simulink model "main1"  (Simulink 10.0)
settings: Solver=ode45  StartTime=0.0  StopTime=0.5  RelTol=1e-3  EnableMultiTasking=on
undefined symbols (not defined in the file): D1, Delta, DiscIntNeverNeededParam, Hydride, Metal, Nickel
libraries: elec_lib x216, powerlib x83, fl_lib x9, powerlib_extras x8, simulink x3, nesl_utility x2, electricdrivelib x1
(part 2 of 2)

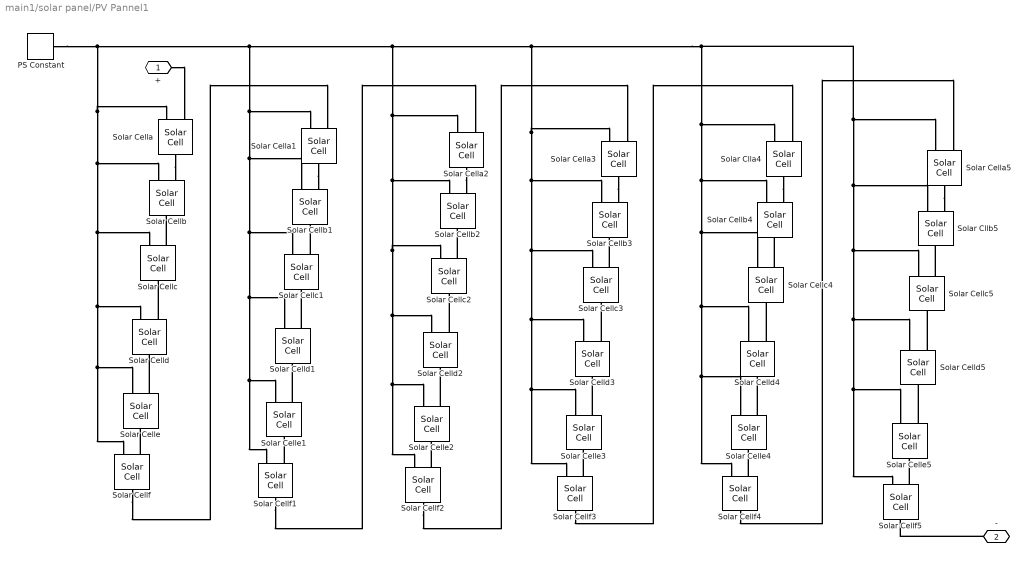
== system main1/solar panel/PV Pannel1 ==
  PS Constant : fl_lib/Physical Signals/Sources/PS Constant  SystemSampleTime=-1  constant=687  LocalVarLogging=[]
  Solar Cella{,1..3,5} (5 alike) : elec_lib/Sources/Solar Cell  SystemSampleTime=-1  prm=1  Isc=2.54 A  Voc=21.8 V  Is=1e-6 A  Is2=0 A  Iph=7.34 A  Ir0=1000 W/m^2  ec=1.6  N2=2  Rs=5.1e-3 Ohm  Rp=Inf Ohm  TIPH1=0.65e-3 1/K  EG=1.12 eV  TXIS1=3  TXIS2=3  TRS1=0  TRP1=0  TFIXED=25 C  Tmeas=25 C  LocalVarLogging=[]
      settings: SourceProductName=Simscape Electrical  SourceProductBaseCode=PS
  Solar Cellb{,1..4} (5 alike) : elec_lib/Sources/Solar Cell  SystemSampleTime=-1  prm=1  Isc=2.54 A  Voc=21.8 V  Is=1e-6 A  Is2=0 A  Iph=7.34 A  Ir0=1000 W/m^2  ec=1.6  N2=2  Rs=5.1e-3 Ohm  Rp=Inf Ohm  TIPH1=0.65e-3 1/K  EG=1.12 eV  TXIS1=3  TXIS2=3  TRS1=0  TRP1=0  TFIXED=25 C  Tmeas=25 C  LocalVarLogging=[]
      settings: SourceProductName=Simscape Electrical  SourceProductBaseCode=PS
  Solar Cellc{,1..5} (6 alike) : elec_lib/Sources/Solar Cell  SystemSampleTime=-1  prm=1  Isc=2.54 A  Voc=21.8 V  Is=1e-6 A  Is2=0 A  Iph=7.34 A  Ir0=1000 W/m^2  ec=1.6  N2=2  Rs=5.1e-3 Ohm  Rp=Inf Ohm  TIPH1=0.65e-3 1/K  EG=1.12 eV  TXIS1=3  TXIS2=3  TRS1=0  TRP1=0  TFIXED=25 C  Tmeas=25 C  LocalVarLogging=[]
      settings: SourceProductName=Simscape Electrical  SourceProductBaseCode=PS
  Solar Celld{,1..5} (6 alike) : elec_lib/Sources/Solar Cell  SystemSampleTime=-1  prm=1  Isc=2.54 A  Voc=21.8 V  Is=1e-6 A  Is2=0 A  Iph=7.34 A  Ir0=1000 W/m^2  ec=1.6  N2=2  Rs=5.1e-3 Ohm  Rp=Inf Ohm  TIPH1=0.65e-3 1/K  EG=1.12 eV  TXIS1=3  TXIS2=3  TRS1=0  TRP1=0  TFIXED=25 C  Tmeas=25 C  LocalVarLogging=[]
      settings: SourceProductName=Simscape Electrical  SourceProductBaseCode=PS
  Solar Celle{,1..5} (6 alike) : elec_lib/Sources/Solar Cell  SystemSampleTime=-1  prm=1  Isc=2.54 A  Voc=21.8 V  Is=1e-6 A  Is2=0 A  Iph=7.34 A  Ir0=1000 W/m^2  ec=1.6  N2=2  Rs=5.1e-3 Ohm  Rp=Inf Ohm  TIPH1=0.65e-3 1/K  EG=1.12 eV  TXIS1=3  TXIS2=3  TRS1=0  TRP1=0  TFIXED=25 C  Tmeas=25 C  LocalVarLogging=[]
      settings: SourceProductName=Simscape Electrical  SourceProductBaseCode=PS
  Solar Cellf{,1..5} (6 alike) : elec_lib/Sources/Solar Cell  SystemSampleTime=-1  prm=1  Isc=2.54 A  Voc=21.8 V  Is=1e-6 A  Is2=0 A  Iph=7.34 A  Ir0=1000 W/m^2  ec=1.6  N2=2  Rs=5.1e-3 Ohm  Rp=Inf Ohm  TIPH1=0.65e-3 1/K  EG=1.12 eV  TXIS1=3  TXIS2=3  TRS1=0  TRP1=0  TFIXED=25 C  Tmeas=25 C  LocalVarLogging=[]
      settings: SourceProductName=Simscape Electrical  SourceProductBaseCode=PS
  Solar Clla4 : elec_lib/Sources/Solar Cell  SystemSampleTime=-1  prm=1  Isc=2.54 A  Voc=21.8 V  Is=1e-6 A  Is2=0 A  Iph=7.34 A  Ir0=1000 W/m^2  ec=1.6  N2=2  Rs=5.1e-3 Ohm  Rp=Inf Ohm  TIPH1=0.65e-3 1/K  EG=1.12 eV  TXIS1=3  TXIS2=3  TRS1=0  TRP1=0  TFIXED=25 C  Tmeas=25 C  LocalVarLogging=[]
      settings: SourceProductName=Simscape Electrical  SourceProductBaseCode=PS
  Solar Cllb5 : elec_lib/Sources/Solar Cell  SystemSampleTime=-1  prm=1  Isc=2.54 A  Voc=21.8 V  Is=1e-6 A  Is2=0 A  Iph=7.34 A  Ir0=1000 W/m^2  ec=1.6  N2=2  Rs=5.1e-3 Ohm  Rp=Inf Ohm  TIPH1=0.65e-3 1/K  EG=1.12 eV  TXIS1=3  TXIS2=3  TRS1=0  TRP1=0  TFIXED=25 C  Tmeas=25 C  LocalVarLogging=[]
      settings: SourceProductName=Simscape Electrical  SourceProductBaseCode=PS
  + : PMIOPort  Side=Left
  - : PMIOPort  Port=2  Side=Left
  connections:
  -/RConn1 -- Solar Cellf5/RConn1
  +/RConn1 -- Solar Cella/LConn2
  Solar Cella3/LConn1 -- Solar Cellb3/LConn1 -- Solar Cellc3/LConn1 -- Solar Celld3/LConn1 -- Solar Celle3/LConn1 -- Solar Cellf3/LConn1 -- Solar Celle2/LConn1 -- Solar Cellf2/LConn1 -- Solar Celld2/LConn1 -- Solar Cellc2/LConn1 -- Solar Cellb2/LConn1 -- Solar Cella2/LConn1 -- Solar Cella1/LConn1 -- Solar Cellb1/LConn1 -- Solar Cellc1/LConn1 -- Solar Celld1/LConn1 -- Solar Celle1/LConn1 -- Solar Cellf1/LConn1 -- Solar Cella/LConn1 -- Solar Cellb/LConn1 -- Solar Cellc/LConn1 -- Solar Celld/LConn1 -- Solar Celle/LConn1 -- Solar Cellf/LConn1 -- PS Constant/RConn1 -- Solar Celle5/LConn1 -- Solar Cellf5/LConn1 -- Solar Celld5/LConn1 -- Solar Cellc5/LConn1 -- Solar Cllb5/LConn1 -- Solar Cella5/LConn1 -- Solar Clla4/LConn1 -- Solar Cellb4/LConn1 -- Solar Cellc4/LConn1 -- Solar Celld4/LConn1 -- Solar Celle4/LConn1 -- Solar Cellf4/LConn1
  Solar Cellf4/RConn1 -- Solar Cella5/LConn2
  Solar Cellf3/RConn1 -- Solar Clla4/LConn2
  Solar Cellf2/RConn1 -- Solar Cella3/LConn2
  Solar Cellf1/RConn1 -- Solar Cella2/LConn2
  Solar Cellf/RConn1 -- Solar Cella1/LConn2
  Solar Cellf5/LConn2 -- Solar Celle5/RConn1
  Solar Celle5/LConn2 -- Solar Celld5/RConn1
  Solar Celld5/LConn2 -- Solar Cellc5/RConn1
  Solar Cellc5/LConn2 -- Solar Cllb5/RConn1
  Solar Cella5/RConn1 -- Solar Cllb5/LConn2
  Solar Cellf4/LConn2 -- Solar Celle4/RConn1
  Solar Celle4/LConn2 -- Solar Celld4/RConn1
  Solar Celld4/LConn2 -- Solar Cellc4/RConn1
  Solar Cellc4/LConn2 -- Solar Cellb4/RConn1
  Solar Clla4/RConn1 -- Solar Cellb4/LConn2
  Solar Cellf3/LConn2 -- Solar Celle3/RConn1
  Solar Celle3/LConn2 -- Solar Celld3/RConn1
  Solar Celld3/LConn2 -- Solar Cellc3/RConn1
  Solar Cellc3/LConn2 -- Solar Cellb3/RConn1
  Solar Cella3/RConn1 -- Solar Cellb3/LConn2
  Solar Cellf2/LConn2 -- Solar Celle2/RConn1
  Solar Celle2/LConn2 -- Solar Celld2/RConn1
  Solar Celld2/LConn2 -- Solar Cellc2/RConn1
  Solar Cellc2/LConn2 -- Solar Cellb2/RConn1
  Solar Cella2/RConn1 -- Solar Cellb2/LConn2
  Solar Cellf1/LConn2 -- Solar Celle1/RConn1
  Solar Celle1/LConn2 -- Solar Celld1/RConn1
  Solar Celld1/LConn2 -- Solar Cellc1/RConn1
  Solar Cellc1/LConn2 -- Solar Cellb1/RConn1
  Solar Cella1/RConn1 -- Solar Cellb1/LConn2
  Solar Cellf/LConn2 -- Solar Celle/RConn1
  Solar Celle/LConn2 -- Solar Celld/RConn1
  Solar Celld/LConn2 -- Solar Cellc/RConn1
  Solar Cellc/LConn2 -- Solar Cellb/RConn1
  Solar Cella/RConn1 -- Solar Cellb/LConn2

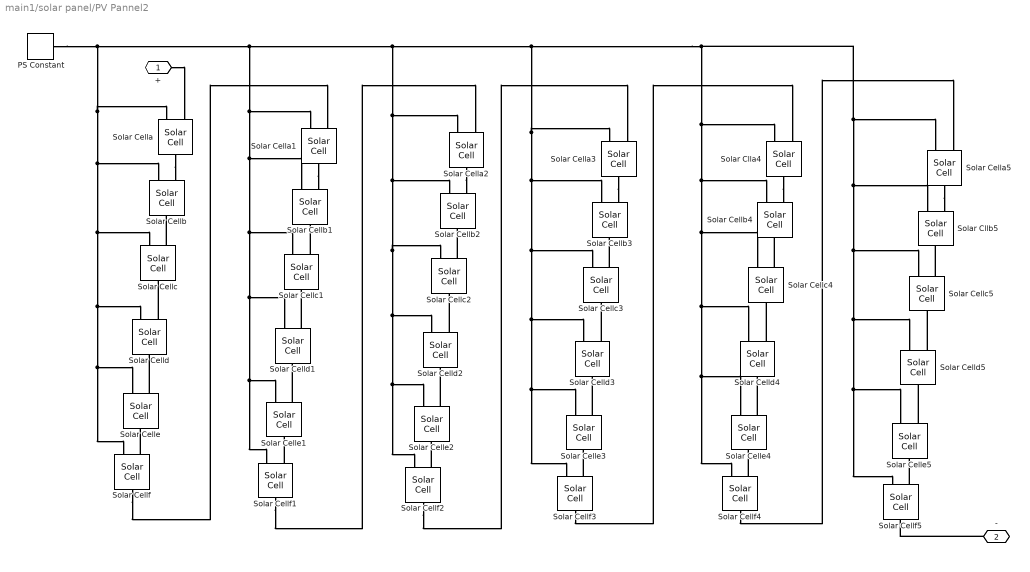
== system main1/solar panel/PV Pannel2 ==
  PS Constant : fl_lib/Physical Signals/Sources/PS Constant  SystemSampleTime=-1  constant=687  LocalVarLogging=[]
  Solar Cella{,1..3,5} (5 alike) : elec_lib/Sources/Solar Cell  SystemSampleTime=-1  prm=1  Isc=2.54 A  Voc=21.8 V  Is=1e-6 A  Is2=0 A  Iph=7.34 A  Ir0=1000 W/m^2  ec=1.6  N2=2  Rs=5.1e-3 Ohm  Rp=Inf Ohm  TIPH1=0.65e-3 1/K  EG=1.12 eV  TXIS1=3  TXIS2=3  TRS1=0  TRP1=0  TFIXED=25 C  Tmeas=25 C  LocalVarLogging=[]
      settings: SourceProductName=Simscape Electrical  SourceProductBaseCode=PS
  Solar Cellb{,1..4} (5 alike) : elec_lib/Sources/Solar Cell  SystemSampleTime=-1  prm=1  Isc=2.54 A  Voc=21.8 V  Is=1e-6 A  Is2=0 A  Iph=7.34 A  Ir0=1000 W/m^2  ec=1.6  N2=2  Rs=5.1e-3 Ohm  Rp=Inf Ohm  TIPH1=0.65e-3 1/K  EG=1.12 eV  TXIS1=3  TXIS2=3  TRS1=0  TRP1=0  TFIXED=25 C  Tmeas=25 C  LocalVarLogging=[]
      settings: SourceProductName=Simscape Electrical  SourceProductBaseCode=PS
  Solar Cellc{,1..5} (6 alike) : elec_lib/Sources/Solar Cell  SystemSampleTime=-1  prm=1  Isc=2.54 A  Voc=21.8 V  Is=1e-6 A  Is2=0 A  Iph=7.34 A  Ir0=1000 W/m^2  ec=1.6  N2=2  Rs=5.1e-3 Ohm  Rp=Inf Ohm  TIPH1=0.65e-3 1/K  EG=1.12 eV  TXIS1=3  TXIS2=3  TRS1=0  TRP1=0  TFIXED=25 C  Tmeas=25 C  LocalVarLogging=[]
      settings: SourceProductName=Simscape Electrical  SourceProductBaseCode=PS
  Solar Celld{,1..5} (6 alike) : elec_lib/Sources/Solar Cell  SystemSampleTime=-1  prm=1  Isc=2.54 A  Voc=21.8 V  Is=1e-6 A  Is2=0 A  Iph=7.34 A  Ir0=1000 W/m^2  ec=1.6  N2=2  Rs=5.1e-3 Ohm  Rp=Inf Ohm  TIPH1=0.65e-3 1/K  EG=1.12 eV  TXIS1=3  TXIS2=3  TRS1=0  TRP1=0  TFIXED=25 C  Tmeas=25 C  LocalVarLogging=[]
      settings: SourceProductName=Simscape Electrical  SourceProductBaseCode=PS
  Solar Celle{,1..5} (6 alike) : elec_lib/Sources/Solar Cell  SystemSampleTime=-1  prm=1  Isc=2.54 A  Voc=21.8 V  Is=1e-6 A  Is2=0 A  Iph=7.34 A  Ir0=1000 W/m^2  ec=1.6  N2=2  Rs=5.1e-3 Ohm  Rp=Inf Ohm  TIPH1=0.65e-3 1/K  EG=1.12 eV  TXIS1=3  TXIS2=3  TRS1=0  TRP1=0  TFIXED=25 C  Tmeas=25 C  LocalVarLogging=[]
      settings: SourceProductName=Simscape Electrical  SourceProductBaseCode=PS
  Solar Cellf{,1..5} (6 alike) : elec_lib/Sources/Solar Cell  SystemSampleTime=-1  prm=1  Isc=2.54 A  Voc=21.8 V  Is=1e-6 A  Is2=0 A  Iph=7.34 A  Ir0=1000 W/m^2  ec=1.6  N2=2  Rs=5.1e-3 Ohm  Rp=Inf Ohm  TIPH1=0.65e-3 1/K  EG=1.12 eV  TXIS1=3  TXIS2=3  TRS1=0  TRP1=0  TFIXED=25 C  Tmeas=25 C  LocalVarLogging=[]
      settings: SourceProductName=Simscape Electrical  SourceProductBaseCode=PS
  Solar Clla4 : elec_lib/Sources/Solar Cell  SystemSampleTime=-1  prm=1  Isc=2.54 A  Voc=21.8 V  Is=1e-6 A  Is2=0 A  Iph=7.34 A  Ir0=1000 W/m^2  ec=1.6  N2=2  Rs=5.1e-3 Ohm  Rp=Inf Ohm  TIPH1=0.65e-3 1/K  EG=1.12 eV  TXIS1=3  TXIS2=3  TRS1=0  TRP1=0  TFIXED=25 C  Tmeas=25 C  LocalVarLogging=[]
      settings: SourceProductName=Simscape Electrical  SourceProductBaseCode=PS
  Solar Cllb5 : elec_lib/Sources/Solar Cell  SystemSampleTime=-1  prm=1  Isc=2.54 A  Voc=21.8 V  Is=1e-6 A  Is2=0 A  Iph=7.34 A  Ir0=1000 W/m^2  ec=1.6  N2=2  Rs=5.1e-3 Ohm  Rp=Inf Ohm  TIPH1=0.65e-3 1/K  EG=1.12 eV  TXIS1=3  TXIS2=3  TRS1=0  TRP1=0  TFIXED=25 C  Tmeas=25 C  LocalVarLogging=[]
      settings: SourceProductName=Simscape Electrical  SourceProductBaseCode=PS
  + : PMIOPort  Side=Left
  - : PMIOPort  Port=2  Side=Left
  connections:
  -/RConn1 -- Solar Cellf5/RConn1
  +/RConn1 -- Solar Cella/LConn2
  Solar Cella3/LConn1 -- Solar Cellb3/LConn1 -- Solar Cellc3/LConn1 -- Solar Celld3/LConn1 -- Solar Celle3/LConn1 -- Solar Cellf3/LConn1 -- Solar Celle2/LConn1 -- Solar Cellf2/LConn1 -- Solar Celld2/LConn1 -- Solar Cellc2/LConn1 -- Solar Cellb2/LConn1 -- Solar Cella2/LConn1 -- Solar Cella1/LConn1 -- Solar Cellb1/LConn1 -- Solar Cellc1/LConn1 -- Solar Celld1/LConn1 -- Solar Celle1/LConn1 -- Solar Cellf1/LConn1 -- Solar Cella/LConn1 -- Solar Cellb/LConn1 -- Solar Cellc/LConn1 -- Solar Celld/LConn1 -- Solar Celle/LConn1 -- Solar Cellf/LConn1 -- PS Constant/RConn1 -- Solar Celle5/LConn1 -- Solar Cellf5/LConn1 -- Solar Celld5/LConn1 -- Solar Cellc5/LConn1 -- Solar Cllb5/LConn1 -- Solar Cella5/LConn1 -- Solar Clla4/LConn1 -- Solar Cellb4/LConn1 -- Solar Cellc4/LConn1 -- Solar Celld4/LConn1 -- Solar Celle4/LConn1 -- Solar Cellf4/LConn1
  Solar Cellf4/RConn1 -- Solar Cella5/LConn2
  Solar Cellf3/RConn1 -- Solar Clla4/LConn2
  Solar Cellf2/RConn1 -- Solar Cella3/LConn2
  Solar Cellf1/RConn1 -- Solar Cella2/LConn2
  Solar Cellf/RConn1 -- Solar Cella1/LConn2
  Solar Cellf5/LConn2 -- Solar Celle5/RConn1
  Solar Celle5/LConn2 -- Solar Celld5/RConn1
  Solar Celld5/LConn2 -- Solar Cellc5/RConn1
  Solar Cellc5/LConn2 -- Solar Cllb5/RConn1
  Solar Cella5/RConn1 -- Solar Cllb5/LConn2
  Solar Cellf4/LConn2 -- Solar Celle4/RConn1
  Solar Celle4/LConn2 -- Solar Celld4/RConn1
  Solar Celld4/LConn2 -- Solar Cellc4/RConn1
  Solar Cellc4/LConn2 -- Solar Cellb4/RConn1
  Solar Clla4/RConn1 -- Solar Cellb4/LConn2
  Solar Cellf3/LConn2 -- Solar Celle3/RConn1
  Solar Celle3/LConn2 -- Solar Celld3/RConn1
  Solar Celld3/LConn2 -- Solar Cellc3/RConn1
  Solar Cellc3/LConn2 -- Solar Cellb3/RConn1
  Solar Cella3/RConn1 -- Solar Cellb3/LConn2
  Solar Cellf2/LConn2 -- Solar Celle2/RConn1
  Solar Celle2/LConn2 -- Solar Celld2/RConn1
  Solar Celld2/LConn2 -- Solar Cellc2/RConn1
  Solar Cellc2/LConn2 -- Solar Cellb2/RConn1
  Solar Cella2/RConn1 -- Solar Cellb2/LConn2
  Solar Cellf1/LConn2 -- Solar Celle1/RConn1
  Solar Celle1/LConn2 -- Solar Celld1/RConn1
  Solar Celld1/LConn2 -- Solar Cellc1/RConn1
  Solar Cellc1/LConn2 -- Solar Cellb1/RConn1
  Solar Cella1/RConn1 -- Solar Cellb1/LConn2
  Solar Cellf/LConn2 -- Solar Celle/RConn1
  Solar Celle/LConn2 -- Solar Celld/RConn1
  Solar Celld/LConn2 -- Solar Cellc/RConn1
  Solar Cellc/LConn2 -- Solar Cellb/RConn1
  Solar Cella/RConn1 -- Solar Cellb/LConn2

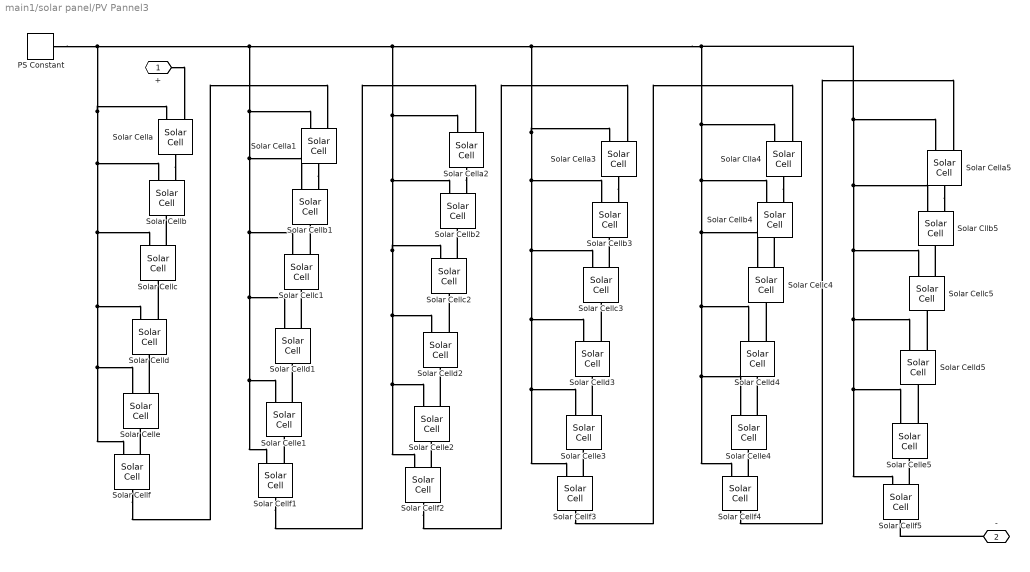
== system main1/solar panel/PV Pannel3 ==
  PS Constant : fl_lib/Physical Signals/Sources/PS Constant  SystemSampleTime=-1  constant=687  LocalVarLogging=[]
  Solar Cella{,1..3,5} (5 alike) : elec_lib/Sources/Solar Cell  SystemSampleTime=-1  prm=1  Isc=2.54 A  Voc=21.8 V  Is=1e-6 A  Is2=0 A  Iph=7.34 A  Ir0=1000 W/m^2  ec=1.6  N2=2  Rs=5.1e-3 Ohm  Rp=Inf Ohm  TIPH1=0.65e-3 1/K  EG=1.12 eV  TXIS1=3  TXIS2=3  TRS1=0  TRP1=0  TFIXED=25 C  Tmeas=25 C  LocalVarLogging=[]
      settings: SourceProductName=Simscape Electrical  SourceProductBaseCode=PS
  Solar Cellb{,1..4} (5 alike) : elec_lib/Sources/Solar Cell  SystemSampleTime=-1  prm=1  Isc=2.54 A  Voc=21.8 V  Is=1e-6 A  Is2=0 A  Iph=7.34 A  Ir0=1000 W/m^2  ec=1.6  N2=2  Rs=5.1e-3 Ohm  Rp=Inf Ohm  TIPH1=0.65e-3 1/K  EG=1.12 eV  TXIS1=3  TXIS2=3  TRS1=0  TRP1=0  TFIXED=25 C  Tmeas=25 C  LocalVarLogging=[]
      settings: SourceProductName=Simscape Electrical  SourceProductBaseCode=PS
  Solar Cellc{,1..5} (6 alike) : elec_lib/Sources/Solar Cell  SystemSampleTime=-1  prm=1  Isc=2.54 A  Voc=21.8 V  Is=1e-6 A  Is2=0 A  Iph=7.34 A  Ir0=1000 W/m^2  ec=1.6  N2=2  Rs=5.1e-3 Ohm  Rp=Inf Ohm  TIPH1=0.65e-3 1/K  EG=1.12 eV  TXIS1=3  TXIS2=3  TRS1=0  TRP1=0  TFIXED=25 C  Tmeas=25 C  LocalVarLogging=[]
      settings: SourceProductName=Simscape Electrical  SourceProductBaseCode=PS
  Solar Celld{,1..5} (6 alike) : elec_lib/Sources/Solar Cell  SystemSampleTime=-1  prm=1  Isc=2.54 A  Voc=21.8 V  Is=1e-6 A  Is2=0 A  Iph=7.34 A  Ir0=1000 W/m^2  ec=1.6  N2=2  Rs=5.1e-3 Ohm  Rp=Inf Ohm  TIPH1=0.65e-3 1/K  EG=1.12 eV  TXIS1=3  TXIS2=3  TRS1=0  TRP1=0  TFIXED=25 C  Tmeas=25 C  LocalVarLogging=[]
      settings: SourceProductName=Simscape Electrical  SourceProductBaseCode=PS
  Solar Celle{,1..5} (6 alike) : elec_lib/Sources/Solar Cell  SystemSampleTime=-1  prm=1  Isc=2.54 A  Voc=21.8 V  Is=1e-6 A  Is2=0 A  Iph=7.34 A  Ir0=1000 W/m^2  ec=1.6  N2=2  Rs=5.1e-3 Ohm  Rp=Inf Ohm  TIPH1=0.65e-3 1/K  EG=1.12 eV  TXIS1=3  TXIS2=3  TRS1=0  TRP1=0  TFIXED=25 C  Tmeas=25 C  LocalVarLogging=[]
      settings: SourceProductName=Simscape Electrical  SourceProductBaseCode=PS
  Solar Cellf{,1..5} (6 alike) : elec_lib/Sources/Solar Cell  SystemSampleTime=-1  prm=1  Isc=2.54 A  Voc=21.8 V  Is=1e-6 A  Is2=0 A  Iph=7.34 A  Ir0=1000 W/m^2  ec=1.6  N2=2  Rs=5.1e-3 Ohm  Rp=Inf Ohm  TIPH1=0.65e-3 1/K  EG=1.12 eV  TXIS1=3  TXIS2=3  TRS1=0  TRP1=0  TFIXED=25 C  Tmeas=25 C  LocalVarLogging=[]
      settings: SourceProductName=Simscape Electrical  SourceProductBaseCode=PS
  Solar Clla4 : elec_lib/Sources/Solar Cell  SystemSampleTime=-1  prm=1  Isc=2.54 A  Voc=21.8 V  Is=1e-6 A  Is2=0 A  Iph=7.34 A  Ir0=1000 W/m^2  ec=1.6  N2=2  Rs=5.1e-3 Ohm  Rp=Inf Ohm  TIPH1=0.65e-3 1/K  EG=1.12 eV  TXIS1=3  TXIS2=3  TRS1=0  TRP1=0  TFIXED=25 C  Tmeas=25 C  LocalVarLogging=[]
      settings: SourceProductName=Simscape Electrical  SourceProductBaseCode=PS
  Solar Cllb5 : elec_lib/Sources/Solar Cell  SystemSampleTime=-1  prm=1  Isc=2.54 A  Voc=21.8 V  Is=1e-6 A  Is2=0 A  Iph=7.34 A  Ir0=1000 W/m^2  ec=1.6  N2=2  Rs=5.1e-3 Ohm  Rp=Inf Ohm  TIPH1=0.65e-3 1/K  EG=1.12 eV  TXIS1=3  TXIS2=3  TRS1=0  TRP1=0  TFIXED=25 C  Tmeas=25 C  LocalVarLogging=[]
      settings: SourceProductName=Simscape Electrical  SourceProductBaseCode=PS
  + : PMIOPort  Side=Left
  - : PMIOPort  Port=2  Side=Left
  connections:
  -/RConn1 -- Solar Cellf5/RConn1
  +/RConn1 -- Solar Cella/LConn2
  Solar Cella3/LConn1 -- Solar Cellb3/LConn1 -- Solar Cellc3/LConn1 -- Solar Celld3/LConn1 -- Solar Celle3/LConn1 -- Solar Cellf3/LConn1 -- Solar Celle2/LConn1 -- Solar Cellf2/LConn1 -- Solar Celld2/LConn1 -- Solar Cellc2/LConn1 -- Solar Cellb2/LConn1 -- Solar Cella2/LConn1 -- Solar Cella1/LConn1 -- Solar Cellb1/LConn1 -- Solar Cellc1/LConn1 -- Solar Celld1/LConn1 -- Solar Celle1/LConn1 -- Solar Cellf1/LConn1 -- Solar Cella/LConn1 -- Solar Cellb/LConn1 -- Solar Cellc/LConn1 -- Solar Celld/LConn1 -- Solar Celle/LConn1 -- Solar Cellf/LConn1 -- PS Constant/RConn1 -- Solar Celle5/LConn1 -- Solar Cellf5/LConn1 -- Solar Celld5/LConn1 -- Solar Cellc5/LConn1 -- Solar Cllb5/LConn1 -- Solar Cella5/LConn1 -- Solar Clla4/LConn1 -- Solar Cellb4/LConn1 -- Solar Cellc4/LConn1 -- Solar Celld4/LConn1 -- Solar Celle4/LConn1 -- Solar Cellf4/LConn1
  Solar Cellf4/RConn1 -- Solar Cella5/LConn2
  Solar Cellf3/RConn1 -- Solar Clla4/LConn2
  Solar Cellf2/RConn1 -- Solar Cella3/LConn2
  Solar Cellf1/RConn1 -- Solar Cella2/LConn2
  Solar Cellf/RConn1 -- Solar Cella1/LConn2
  Solar Cellf5/LConn2 -- Solar Celle5/RConn1
  Solar Celle5/LConn2 -- Solar Celld5/RConn1
  Solar Celld5/LConn2 -- Solar Cellc5/RConn1
  Solar Cellc5/LConn2 -- Solar Cllb5/RConn1
  Solar Cella5/RConn1 -- Solar Cllb5/LConn2
  Solar Cellf4/LConn2 -- Solar Celle4/RConn1
  Solar Celle4/LConn2 -- Solar Celld4/RConn1
  Solar Celld4/LConn2 -- Solar Cellc4/RConn1
  Solar Cellc4/LConn2 -- Solar Cellb4/RConn1
  Solar Clla4/RConn1 -- Solar Cellb4/LConn2
  Solar Cellf3/LConn2 -- Solar Celle3/RConn1
  Solar Celle3/LConn2 -- Solar Celld3/RConn1
  Solar Celld3/LConn2 -- Solar Cellc3/RConn1
  Solar Cellc3/LConn2 -- Solar Cellb3/RConn1
  Solar Cella3/RConn1 -- Solar Cellb3/LConn2
  Solar Cellf2/LConn2 -- Solar Celle2/RConn1
  Solar Celle2/LConn2 -- Solar Celld2/RConn1
  Solar Celld2/LConn2 -- Solar Cellc2/RConn1
  Solar Cellc2/LConn2 -- Solar Cellb2/RConn1
  Solar Cella2/RConn1 -- Solar Cellb2/LConn2
  Solar Cellf1/LConn2 -- Solar Celle1/RConn1
  Solar Celle1/LConn2 -- Solar Celld1/RConn1
  Solar Celld1/LConn2 -- Solar Cellc1/RConn1
  Solar Cellc1/LConn2 -- Solar Cellb1/RConn1
  Solar Cella1/RConn1 -- Solar Cellb1/LConn2
  Solar Cellf/LConn2 -- Solar Celle/RConn1
  Solar Celle/LConn2 -- Solar Celld/RConn1
  Solar Celld/LConn2 -- Solar Cellc/RConn1
  Solar Cellc/LConn2 -- Solar Cellb/RConn1
  Solar Cella/RConn1 -- Solar Cellb/LConn2

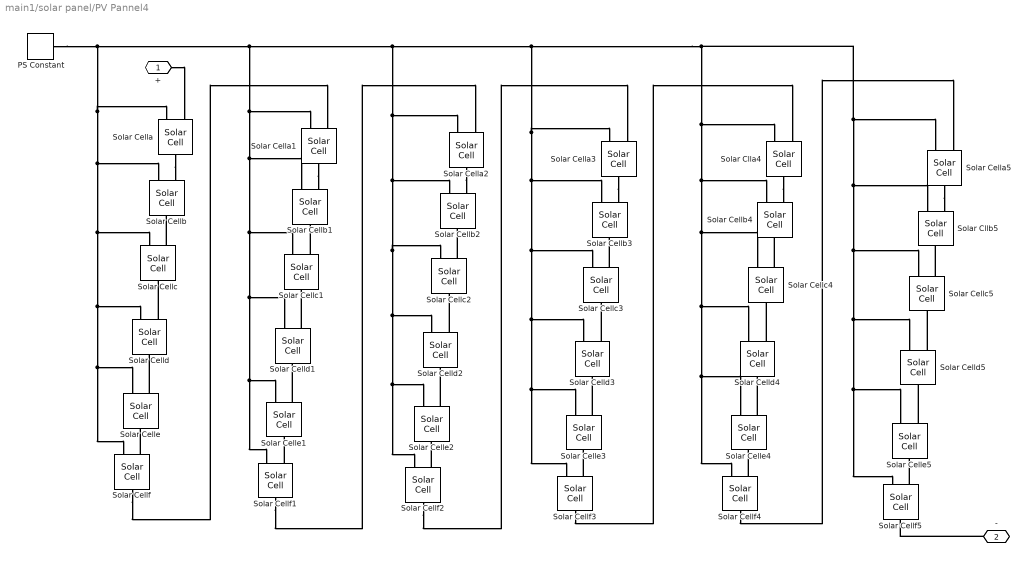
== system main1/solar panel/PV Pannel4 ==
  PS Constant : fl_lib/Physical Signals/Sources/PS Constant  SystemSampleTime=-1  constant=687  LocalVarLogging=[]
  Solar Cella{,1..3,5} (5 alike) : elec_lib/Sources/Solar Cell  SystemSampleTime=-1  prm=1  Isc=2.54 A  Voc=21.8 V  Is=1e-6 A  Is2=0 A  Iph=7.34 A  Ir0=1000 W/m^2  ec=1.6  N2=2  Rs=5.1e-3 Ohm  Rp=Inf Ohm  TIPH1=0.65e-3 1/K  EG=1.12 eV  TXIS1=3  TXIS2=3  TRS1=0  TRP1=0  TFIXED=25 C  Tmeas=25 C  LocalVarLogging=[]
      settings: SourceProductName=Simscape Electrical  SourceProductBaseCode=PS
  Solar Cellb{,1..4} (5 alike) : elec_lib/Sources/Solar Cell  SystemSampleTime=-1  prm=1  Isc=2.54 A  Voc=21.8 V  Is=1e-6 A  Is2=0 A  Iph=7.34 A  Ir0=1000 W/m^2  ec=1.6  N2=2  Rs=5.1e-3 Ohm  Rp=Inf Ohm  TIPH1=0.65e-3 1/K  EG=1.12 eV  TXIS1=3  TXIS2=3  TRS1=0  TRP1=0  TFIXED=25 C  Tmeas=25 C  LocalVarLogging=[]
      settings: SourceProductName=Simscape Electrical  SourceProductBaseCode=PS
  Solar Cellc{,1..5} (6 alike) : elec_lib/Sources/Solar Cell  SystemSampleTime=-1  prm=1  Isc=2.54 A  Voc=21.8 V  Is=1e-6 A  Is2=0 A  Iph=7.34 A  Ir0=1000 W/m^2  ec=1.6  N2=2  Rs=5.1e-3 Ohm  Rp=Inf Ohm  TIPH1=0.65e-3 1/K  EG=1.12 eV  TXIS1=3  TXIS2=3  TRS1=0  TRP1=0  TFIXED=25 C  Tmeas=25 C  LocalVarLogging=[]
      settings: SourceProductName=Simscape Electrical  SourceProductBaseCode=PS
  Solar Celld{,1..5} (6 alike) : elec_lib/Sources/Solar Cell  SystemSampleTime=-1  prm=1  Isc=2.54 A  Voc=21.8 V  Is=1e-6 A  Is2=0 A  Iph=7.34 A  Ir0=1000 W/m^2  ec=1.6  N2=2  Rs=5.1e-3 Ohm  Rp=Inf Ohm  TIPH1=0.65e-3 1/K  EG=1.12 eV  TXIS1=3  TXIS2=3  TRS1=0  TRP1=0  TFIXED=25 C  Tmeas=25 C  LocalVarLogging=[]
      settings: SourceProductName=Simscape Electrical  SourceProductBaseCode=PS
  Solar Celle{,1..5} (6 alike) : elec_lib/Sources/Solar Cell  SystemSampleTime=-1  prm=1  Isc=2.54 A  Voc=21.8 V  Is=1e-6 A  Is2=0 A  Iph=7.34 A  Ir0=1000 W/m^2  ec=1.6  N2=2  Rs=5.1e-3 Ohm  Rp=Inf Ohm  TIPH1=0.65e-3 1/K  EG=1.12 eV  TXIS1=3  TXIS2=3  TRS1=0  TRP1=0  TFIXED=25 C  Tmeas=25 C  LocalVarLogging=[]
      settings: SourceProductName=Simscape Electrical  SourceProductBaseCode=PS
  Solar Cellf{,1..5} (6 alike) : elec_lib/Sources/Solar Cell  SystemSampleTime=-1  prm=1  Isc=2.54 A  Voc=21.8 V  Is=1e-6 A  Is2=0 A  Iph=7.34 A  Ir0=1000 W/m^2  ec=1.6  N2=2  Rs=5.1e-3 Ohm  Rp=Inf Ohm  TIPH1=0.65e-3 1/K  EG=1.12 eV  TXIS1=3  TXIS2=3  TRS1=0  TRP1=0  TFIXED=25 C  Tmeas=25 C  LocalVarLogging=[]
      settings: SourceProductName=Simscape Electrical  SourceProductBaseCode=PS
  Solar Clla4 : elec_lib/Sources/Solar Cell  SystemSampleTime=-1  prm=1  Isc=2.54 A  Voc=21.8 V  Is=1e-6 A  Is2=0 A  Iph=7.34 A  Ir0=1000 W/m^2  ec=1.6  N2=2  Rs=5.1e-3 Ohm  Rp=Inf Ohm  TIPH1=0.65e-3 1/K  EG=1.12 eV  TXIS1=3  TXIS2=3  TRS1=0  TRP1=0  TFIXED=25 C  Tmeas=25 C  LocalVarLogging=[]
      settings: SourceProductName=Simscape Electrical  SourceProductBaseCode=PS
  Solar Cllb5 : elec_lib/Sources/Solar Cell  SystemSampleTime=-1  prm=1  Isc=2.54 A  Voc=21.8 V  Is=1e-6 A  Is2=0 A  Iph=7.34 A  Ir0=1000 W/m^2  ec=1.6  N2=2  Rs=5.1e-3 Ohm  Rp=Inf Ohm  TIPH1=0.65e-3 1/K  EG=1.12 eV  TXIS1=3  TXIS2=3  TRS1=0  TRP1=0  TFIXED=25 C  Tmeas=25 C  LocalVarLogging=[]
      settings: SourceProductName=Simscape Electrical  SourceProductBaseCode=PS
  + : PMIOPort  Side=Left
  - : PMIOPort  Port=2  Side=Left
  connections:
  -/RConn1 -- Solar Cellf5/RConn1
  +/RConn1 -- Solar Cella/LConn2
  Solar Cella3/LConn1 -- Solar Cellb3/LConn1 -- Solar Cellc3/LConn1 -- Solar Celld3/LConn1 -- Solar Celle3/LConn1 -- Solar Cellf3/LConn1 -- Solar Celle2/LConn1 -- Solar Cellf2/LConn1 -- Solar Celld2/LConn1 -- Solar Cellc2/LConn1 -- Solar Cellb2/LConn1 -- Solar Cella2/LConn1 -- Solar Cella1/LConn1 -- Solar Cellb1/LConn1 -- Solar Cellc1/LConn1 -- Solar Celld1/LConn1 -- Solar Celle1/LConn1 -- Solar Cellf1/LConn1 -- Solar Cella/LConn1 -- Solar Cellb/LConn1 -- Solar Cellc/LConn1 -- Solar Celld/LConn1 -- Solar Celle/LConn1 -- Solar Cellf/LConn1 -- PS Constant/RConn1 -- Solar Celle5/LConn1 -- Solar Cellf5/LConn1 -- Solar Celld5/LConn1 -- Solar Cellc5/LConn1 -- Solar Cllb5/LConn1 -- Solar Cella5/LConn1 -- Solar Clla4/LConn1 -- Solar Cellb4/LConn1 -- Solar Cellc4/LConn1 -- Solar Celld4/LConn1 -- Solar Celle4/LConn1 -- Solar Cellf4/LConn1
  Solar Cellf4/RConn1 -- Solar Cella5/LConn2
  Solar Cellf3/RConn1 -- Solar Clla4/LConn2
  Solar Cellf2/RConn1 -- Solar Cella3/LConn2
  Solar Cellf1/RConn1 -- Solar Cella2/LConn2
  Solar Cellf/RConn1 -- Solar Cella1/LConn2
  Solar Cellf5/LConn2 -- Solar Celle5/RConn1
  Solar Celle5/LConn2 -- Solar Celld5/RConn1
  Solar Celld5/LConn2 -- Solar Cellc5/RConn1
  Solar Cellc5/LConn2 -- Solar Cllb5/RConn1
  Solar Cella5/RConn1 -- Solar Cllb5/LConn2
  Solar Cellf4/LConn2 -- Solar Celle4/RConn1
  Solar Celle4/LConn2 -- Solar Celld4/RConn1
  Solar Celld4/LConn2 -- Solar Cellc4/RConn1
  Solar Cellc4/LConn2 -- Solar Cellb4/RConn1
  Solar Clla4/RConn1 -- Solar Cellb4/LConn2
  Solar Cellf3/LConn2 -- Solar Celle3/RConn1
  Solar Celle3/LConn2 -- Solar Celld3/RConn1
  Solar Celld3/LConn2 -- Solar Cellc3/RConn1
  Solar Cellc3/LConn2 -- Solar Cellb3/RConn1
  Solar Cella3/RConn1 -- Solar Cellb3/LConn2
  Solar Cellf2/LConn2 -- Solar Celle2/RConn1
  Solar Celle2/LConn2 -- Solar Celld2/RConn1
  Solar Celld2/LConn2 -- Solar Cellc2/RConn1
  Solar Cellc2/LConn2 -- Solar Cellb2/RConn1
  Solar Cella2/RConn1 -- Solar Cellb2/LConn2
  Solar Cellf1/LConn2 -- Solar Celle1/RConn1
  Solar Celle1/LConn2 -- Solar Celld1/RConn1
  Solar Celld1/LConn2 -- Solar Cellc1/RConn1
  Solar Cellc1/LConn2 -- Solar Cellb1/RConn1
  Solar Cella1/RConn1 -- Solar Cellb1/LConn2
  Solar Cellf/LConn2 -- Solar Celle/RConn1
  Solar Celle/LConn2 -- Solar Celld/RConn1
  Solar Celld/LConn2 -- Solar Cellc/RConn1
  Solar Cellc/LConn2 -- Solar Cellb/RConn1
  Solar Cella/RConn1 -- Solar Cellb/LConn2

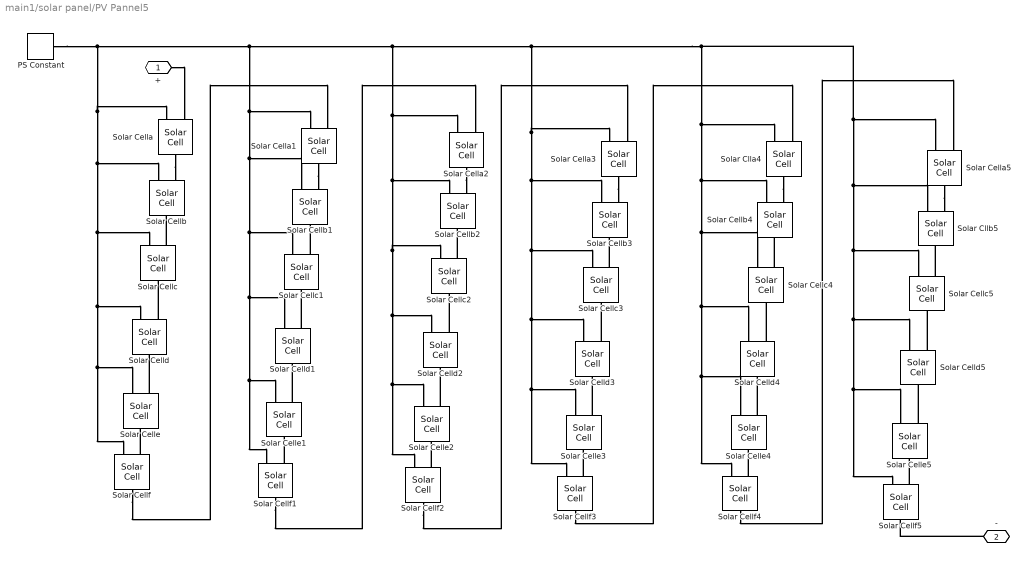
== system main1/solar panel/PV Pannel5 ==
  PS Constant : fl_lib/Physical Signals/Sources/PS Constant  SystemSampleTime=-1  constant=687  LocalVarLogging=[]
  Solar Cella{,1..3,5} (5 alike) : elec_lib/Sources/Solar Cell  SystemSampleTime=-1  prm=1  Isc=2.54 A  Voc=21.8 V  Is=1e-6 A  Is2=0 A  Iph=7.34 A  Ir0=1000 W/m^2  ec=1.6  N2=2  Rs=5.1e-3 Ohm  Rp=Inf Ohm  TIPH1=0.65e-3 1/K  EG=1.12 eV  TXIS1=3  TXIS2=3  TRS1=0  TRP1=0  TFIXED=25 C  Tmeas=25 C  LocalVarLogging=[]
      settings: SourceProductName=Simscape Electrical  SourceProductBaseCode=PS
  Solar Cellb{,1..4} (5 alike) : elec_lib/Sources/Solar Cell  SystemSampleTime=-1  prm=1  Isc=2.54 A  Voc=21.8 V  Is=1e-6 A  Is2=0 A  Iph=7.34 A  Ir0=1000 W/m^2  ec=1.6  N2=2  Rs=5.1e-3 Ohm  Rp=Inf Ohm  TIPH1=0.65e-3 1/K  EG=1.12 eV  TXIS1=3  TXIS2=3  TRS1=0  TRP1=0  TFIXED=25 C  Tmeas=25 C  LocalVarLogging=[]
      settings: SourceProductName=Simscape Electrical  SourceProductBaseCode=PS
  Solar Cellc{,1..5} (6 alike) : elec_lib/Sources/Solar Cell  SystemSampleTime=-1  prm=1  Isc=2.54 A  Voc=21.8 V  Is=1e-6 A  Is2=0 A  Iph=7.34 A  Ir0=1000 W/m^2  ec=1.6  N2=2  Rs=5.1e-3 Ohm  Rp=Inf Ohm  TIPH1=0.65e-3 1/K  EG=1.12 eV  TXIS1=3  TXIS2=3  TRS1=0  TRP1=0  TFIXED=25 C  Tmeas=25 C  LocalVarLogging=[]
      settings: SourceProductName=Simscape Electrical  SourceProductBaseCode=PS
  Solar Celld{,1..5} (6 alike) : elec_lib/Sources/Solar Cell  SystemSampleTime=-1  prm=1  Isc=2.54 A  Voc=21.8 V  Is=1e-6 A  Is2=0 A  Iph=7.34 A  Ir0=1000 W/m^2  ec=1.6  N2=2  Rs=5.1e-3 Ohm  Rp=Inf Ohm  TIPH1=0.65e-3 1/K  EG=1.12 eV  TXIS1=3  TXIS2=3  TRS1=0  TRP1=0  TFIXED=25 C  Tmeas=25 C  LocalVarLogging=[]
      settings: SourceProductName=Simscape Electrical  SourceProductBaseCode=PS
  Solar Celle{,1..5} (6 alike) : elec_lib/Sources/Solar Cell  SystemSampleTime=-1  prm=1  Isc=2.54 A  Voc=21.8 V  Is=1e-6 A  Is2=0 A  Iph=7.34 A  Ir0=1000 W/m^2  ec=1.6  N2=2  Rs=5.1e-3 Ohm  Rp=Inf Ohm  TIPH1=0.65e-3 1/K  EG=1.12 eV  TXIS1=3  TXIS2=3  TRS1=0  TRP1=0  TFIXED=25 C  Tmeas=25 C  LocalVarLogging=[]
      settings: SourceProductName=Simscape Electrical  SourceProductBaseCode=PS
  Solar Cellf{,1..5} (6 alike) : elec_lib/Sources/Solar Cell  SystemSampleTime=-1  prm=1  Isc=2.54 A  Voc=21.8 V  Is=1e-6 A  Is2=0 A  Iph=7.34 A  Ir0=1000 W/m^2  ec=1.6  N2=2  Rs=5.1e-3 Ohm  Rp=Inf Ohm  TIPH1=0.65e-3 1/K  EG=1.12 eV  TXIS1=3  TXIS2=3  TRS1=0  TRP1=0  TFIXED=25 C  Tmeas=25 C  LocalVarLogging=[]
      settings: SourceProductName=Simscape Electrical  SourceProductBaseCode=PS
  Solar Clla4 : elec_lib/Sources/Solar Cell  SystemSampleTime=-1  prm=1  Isc=2.54 A  Voc=21.8 V  Is=1e-6 A  Is2=0 A  Iph=7.34 A  Ir0=1000 W/m^2  ec=1.6  N2=2  Rs=5.1e-3 Ohm  Rp=Inf Ohm  TIPH1=0.65e-3 1/K  EG=1.12 eV  TXIS1=3  TXIS2=3  TRS1=0  TRP1=0  TFIXED=25 C  Tmeas=25 C  LocalVarLogging=[]
      settings: SourceProductName=Simscape Electrical  SourceProductBaseCode=PS
  Solar Cllb5 : elec_lib/Sources/Solar Cell  SystemSampleTime=-1  prm=1  Isc=2.54 A  Voc=21.8 V  Is=1e-6 A  Is2=0 A  Iph=7.34 A  Ir0=1000 W/m^2  ec=1.6  N2=2  Rs=5.1e-3 Ohm  Rp=Inf Ohm  TIPH1=0.65e-3 1/K  EG=1.12 eV  TXIS1=3  TXIS2=3  TRS1=0  TRP1=0  TFIXED=25 C  Tmeas=25 C  LocalVarLogging=[]
      settings: SourceProductName=Simscape Electrical  SourceProductBaseCode=PS
  + : PMIOPort  Side=Left
  - : PMIOPort  Port=2  Side=Left
  connections:
  -/RConn1 -- Solar Cellf5/RConn1
  +/RConn1 -- Solar Cella/LConn2
  Solar Cella3/LConn1 -- Solar Cellb3/LConn1 -- Solar Cellc3/LConn1 -- Solar Celld3/LConn1 -- Solar Celle3/LConn1 -- Solar Cellf3/LConn1 -- Solar Celle2/LConn1 -- Solar Cellf2/LConn1 -- Solar Celld2/LConn1 -- Solar Cellc2/LConn1 -- Solar Cellb2/LConn1 -- Solar Cella2/LConn1 -- Solar Cella1/LConn1 -- Solar Cellb1/LConn1 -- Solar Cellc1/LConn1 -- Solar Celld1/LConn1 -- Solar Celle1/LConn1 -- Solar Cellf1/LConn1 -- Solar Cella/LConn1 -- Solar Cellb/LConn1 -- Solar Cellc/LConn1 -- Solar Celld/LConn1 -- Solar Celle/LConn1 -- Solar Cellf/LConn1 -- PS Constant/RConn1 -- Solar Celle5/LConn1 -- Solar Cellf5/LConn1 -- Solar Celld5/LConn1 -- Solar Cellc5/LConn1 -- Solar Cllb5/LConn1 -- Solar Cella5/LConn1 -- Solar Clla4/LConn1 -- Solar Cellb4/LConn1 -- Solar Cellc4/LConn1 -- Solar Celld4/LConn1 -- Solar Celle4/LConn1 -- Solar Cellf4/LConn1
  Solar Cellf4/RConn1 -- Solar Cella5/LConn2
  Solar Cellf3/RConn1 -- Solar Clla4/LConn2
  Solar Cellf2/RConn1 -- Solar Cella3/LConn2
  Solar Cellf1/RConn1 -- Solar Cella2/LConn2
  Solar Cellf/RConn1 -- Solar Cella1/LConn2
  Solar Cellf5/LConn2 -- Solar Celle5/RConn1
  Solar Celle5/LConn2 -- Solar Celld5/RConn1
  Solar Celld5/LConn2 -- Solar Cellc5/RConn1
  Solar Cellc5/LConn2 -- Solar Cllb5/RConn1
  Solar Cella5/RConn1 -- Solar Cllb5/LConn2
  Solar Cellf4/LConn2 -- Solar Celle4/RConn1
  Solar Celle4/LConn2 -- Solar Celld4/RConn1
  Solar Celld4/LConn2 -- Solar Cellc4/RConn1
  Solar Cellc4/LConn2 -- Solar Cellb4/RConn1
  Solar Clla4/RConn1 -- Solar Cellb4/LConn2
  Solar Cellf3/LConn2 -- Solar Celle3/RConn1
  Solar Celle3/LConn2 -- Solar Celld3/RConn1
  Solar Celld3/LConn2 -- Solar Cellc3/RConn1
  Solar Cellc3/LConn2 -- Solar Cellb3/RConn1
  Solar Cella3/RConn1 -- Solar Cellb3/LConn2
  Solar Cellf2/LConn2 -- Solar Celle2/RConn1
  Solar Celle2/LConn2 -- Solar Celld2/RConn1
  Solar Celld2/LConn2 -- Solar Cellc2/RConn1
  Solar Cellc2/LConn2 -- Solar Cellb2/RConn1
  Solar Cella2/RConn1 -- Solar Cellb2/LConn2
  Solar Cellf1/LConn2 -- Solar Celle1/RConn1
  Solar Celle1/LConn2 -- Solar Celld1/RConn1
  Solar Celld1/LConn2 -- Solar Cellc1/RConn1
  Solar Cellc1/LConn2 -- Solar Cellb1/RConn1
  Solar Cella1/RConn1 -- Solar Cellb1/LConn2
  Solar Cellf/LConn2 -- Solar Celle/RConn1
  Solar Celle/LConn2 -- Solar Celld/RConn1
  Solar Celld/LConn2 -- Solar Cellc/RConn1
  Solar Cellc/LConn2 -- Solar Cellb/RConn1
  Solar Cella/RConn1 -- Solar Cellb/LConn2

== system main1/Subsystem2/Subsystem1/Angle_generator ==
  freq_inp : Inport
  Constant : Constant  Value=360
  Constant1 : Constant  Value=360
  Discrete-Time Integrator1 : DiscreteIntegrator  IntegratorMethod=Integration: Trapezoidal  ExternalReset=rising  SampleTime=5e-6  ICPrevOutput=DiscIntNeverNeededParam  ICPrevScaledInput=DiscIntNeverNeededParam
  Product : Product  SaturateOnIntegerOverflow=on  InputSameDT=on  OutDataTypeStr=Inherit: Same as first input
  Relational Operator : RelationalOperator  RndMeth=Nearest  InputSameDT=on
  Unit Delay : UnitDelay  SampleTime=5e-6
  ramp_out : Outport
  wires:
  Discrete-Time Integrator1/1 -> Relational Operator/1, ramp_out/1
  Constant/1 -> Relational Operator/2
  Relational Operator/1 -> Unit Delay/1
  Unit Delay/1 -> Discrete-Time Integrator1/2
  Constant1/1 -> Product/1
  Product/1 -> Discrete-Time Integrator1/1
  freq_inp/1 -> Product/2

== system main1/Subsystem2/Subsystem1/PQ ==
  carrier_frequency : Inport
  %duty_ratio : Inport  Port=2
  Angle_generator1 : Subsystem
  Gain : Gain  Gain=0.01*360
  Relational Operator1 : RelationalOperator  RndMeth=Nearest  InputSameDT=on
  PWM_signal : Outport
  wires:
  Gain/1 -> Relational Operator1/1
  Angle_generator1/1(ramp_out) -> Relational Operator1/2
  carrier_frequency/1 -> Angle_generator1/1(freq_inp)
  Relational Operator1/1 -> PWM_signal/1
  %duty_ratio/1 -> Gain/1

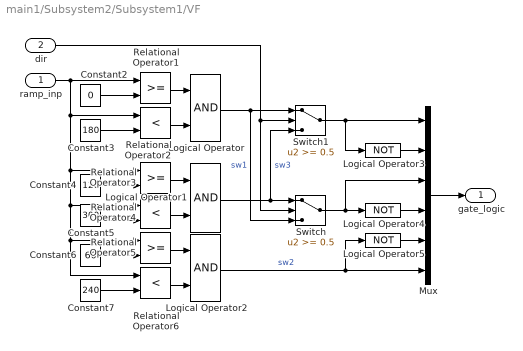
== system main1/Subsystem2/Subsystem1/VF ==
  ramp_inp : Inport
  dir : Inport  Port=2
  Constant2 : Constant  Value=0
  Constant3 : Constant  Value=180
  Constant4 : Constant  Value=120
  Constant5 : Constant  Value=300
  Constant6 : Constant  Value=60
  Constant7 : Constant  Value=240
  Logical Operator : Logic
  Logical Operator1 : Logic
  Logical Operator2 : Logic
  Logical Operator3 : Logic  Operator=NOT
  Logical Operator4 : Logic  Operator=NOT
  Logical Operator5 : Logic  Operator=NOT
  Mux : Mux  Inputs=6
  Relational Operator1 : RelationalOperator  RndMeth=Nearest  InputSameDT=on
  Relational Operator2 : RelationalOperator  Operator=<  RndMeth=Nearest  InputSameDT=on
  Relational Operator3 : RelationalOperator  RndMeth=Nearest  InputSameDT=on
  Relational Operator4 : RelationalOperator  Operator=<  RndMeth=Nearest  InputSameDT=on
  Relational Operator5 : RelationalOperator  RndMeth=Nearest  InputSameDT=on
  Relational Operator6 : RelationalOperator  Operator=<  RndMeth=Nearest  InputSameDT=on
  Switch : Switch  Threshold=0.5  SaturateOnIntegerOverflow=on  InputSameDT=on
  Switch1 : Switch  Threshold=0.5  SaturateOnIntegerOverflow=on  InputSameDT=on
  gate_logic : Outport
  wires:
  Constant4/1 -> Relational Operator3/2
  Constant5/1 -> Relational Operator4/2
  Relational Operator3/1 -> Logical Operator1/1
  Relational Operator4/1 -> Logical Operator1/2
  Constant6/1 -> Relational Operator5/2
  Constant7/1 -> Relational Operator6/2
  Relational Operator5/1 -> Logical Operator2/1
  Relational Operator6/1 -> Logical Operator2/2
  Logical Operator3/1 -> Mux/2
  Logical Operator4/1 -> Mux/4
  Logical Operator5/1 -> Mux/5
  Logical Operator2/1 -> Logical Operator5/1, Mux/6  "sw2"
  Logical Operator/1 -> Switch1/1, Switch/3  "sw1"
  Mux/1 -> gate_logic/1
  Switch1/1 -> Mux/1, Logical Operator3/1
  Switch/1 -> Logical Operator4/1, Mux/3
  dir/1 -> Switch1/2, Switch/2
  Logical Operator1/1 -> Switch/1, Switch1/3  "sw3"
  Constant2/1 -> Relational Operator1/2
  Constant3/1 -> Relational Operator2/2
  Relational Operator1/1 -> Logical Operator/1
  Relational Operator2/1 -> Logical Operator/2
  ramp_inp/1 -> Relational Operator1/1, Relational Operator2/1, Relational Operator3/1, Relational Operator4/1, Relational Operator5/1, Relational Operator6/1

== system main1/Subsystem2/Subsystem1/PQ/Angle_generator1 ==
  freq_inp : Inport
  Constant : Constant  Value=360
  Constant1 : Constant  Value=360
  Discrete-Time Integrator1 : DiscreteIntegrator  IntegratorMethod=Integration: Trapezoidal  ExternalReset=rising  SampleTime=5e-6  ICPrevOutput=DiscIntNeverNeededParam  ICPrevScaledInput=DiscIntNeverNeededParam
  Product : Product  SaturateOnIntegerOverflow=on  InputSameDT=on  OutDataTypeStr=Inherit: Same as first input
  Relational Operator : RelationalOperator  RndMeth=Nearest  InputSameDT=on
  Unit Delay : UnitDelay  SampleTime=5e-6
  ramp_out : Outport
  wires:
  Discrete-Time Integrator1/1 -> Relational Operator/1, ramp_out/1
  Constant/1 -> Relational Operator/2
  Relational Operator/1 -> Unit Delay/1
  Unit Delay/1 -> Discrete-Time Integrator1/2
  Constant1/1 -> Product/1
  Product/1 -> Discrete-Time Integrator1/1
  freq_inp/1 -> Product/2
